simulink model "adaptive_t1"  (R2017a)
settings: Solver=FixedStepAuto  StartTime=0.0  StopTime=8  FixedStep=0.001  RelTol=1e-3
libraries: fuzblock x2
settings Model: Creator=Chaohua Zhao  LastModifiedBy=Chaohua Zhao

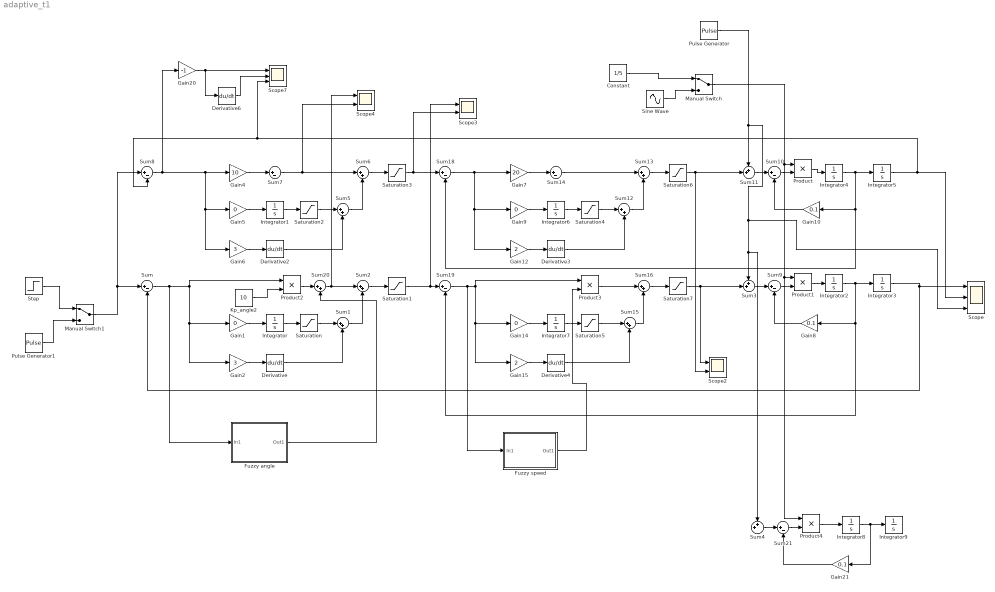
== system adaptive_t1 ==
  Constant : Constant  Value=1/5
  Derivative{,2..4,6} (5 alike) : Derivative
  "Fuzzy angle " : Subsystem
  Fuzzy speed : Subsystem
  Gain{1,5,9,14} (4 alike) : Gain  Gain=0
  Gain10 : Gain  Gain=0.1
  Gain12 : Gain  Gain=2
  Gain15 : Gain  Gain=2
  Gain2 : Gain  Gain=3
  Gain20 : Gain  Gain=-1
  Gain21 : Gain  Gain=0.1
  Gain4 : Gain  Gain=10
  Gain6 : Gain  Gain=3
  Gain7 : Gain  Gain=20
  Gain8 : Gain  Gain=0.1
  Integrator{,1..9} (10 alike) : Integrator
  Kp_angle2 : Constant  Value=10
  Manual Switch : ManualSwitch
  Manual Switch1 : ManualSwitch
  Product{,1..4} (5 alike) : Product
  Pulse Generator : DiscretePulseGenerator  PulseType=Time based  Amplitude=0.1  Period=3  PulseWidth=4  PhaseDelay=5
  Pulse Generator1 : DiscretePulseGenerator  PulseType=Time based  Period=15  PulseWidth=50
  Saturation{,2,4..5} (4 alike) : Saturate
  Saturation1 : Saturate  UpperLimit=100  LowerLimit=-100
  Saturation3 : Saturate  UpperLimit=100  LowerLimit=-100
  Saturation6 : Saturate  UpperLimit=10  LowerLimit=-10
  Saturation7 : Saturate  UpperLimit=10  LowerLimit=-10
  Scope : Scope  NumInputPorts=3
  Scope2 : Scope  NumInputPorts=2
  Scope3 : Scope  NumInputPorts=2
  Scope4 : Scope  NumInputPorts=2
  Scope7 : Scope  NumInputPorts=3
  Sine Wave : Sin  Amplitude=0.4  Bias=0.5  SampleTime=0
  Step : Step  Time=0  After=3  SampleTime=0
  Sum{,7..10,14,18..19,21} (9 alike) : Sum  Inputs=|+-
  Sum{1..2,5..6,12..13,15..16,20} (9 alike) : Sum  Inputs=|++
  Sum11 : Sum  Inputs=++|
  Sum3 : Sum  Inputs=++|
  Sum4 : Sum  Inputs=++|
  wires:
  Integrator3/1 -> Scope/1, Sum/2
  Sum/1 -> "Fuzzy angle "/1(In1), Product2/1, Gain1/1, Gain2/1
  Saturation/1 -> Sum1/1
  Integrator/1 -> Saturation/1
  Gain1/1 -> Integrator/1
  Gain2/1 -> Derivative/1
  Derivative/1 -> Sum1/2
  Sum1/1 -> Sum2/2
  Sum2/1 -> Saturation1/1
  Sum7/1 -> Scope4/2, Sum6/1
  Gain4/1 -> Sum7/1
  Sum6/1 -> Saturation3/1
  Sum5/1 -> Sum6/2
  Derivative2/1 -> Sum5/2
  Gain6/1 -> Derivative2/1
  Gain5/1 -> Integrator1/1
  Integrator1/1 -> Saturation2/1
  Saturation2/1 -> Sum5/1
  Sum8/1 -> Gain20/1, Gain4/1, Gain5/1, Gain6/1
  Integrator5/1 -> Scope7/3, Sum8/2, Scope/2
  Integrator2/1 -> Sum19/2, Gain8/1, Integrator3/1
  Sum3/1 -> Sum9/1
  Integrator4/1 -> Integrator5/1, Sum18/2, Gain10/1
  Sum11/1 -> Sum10/1
  Pulse Generator/1 -> Scope/3, Sum4/1, Sum3/1, Sum11/1
  Sum10/1 -> Product/2
  Product/1 -> Integrator4/1
  Sum9/1 -> Product1/2
  Product1/1 -> Integrator2/1
  Sine Wave/1 -> Manual Switch/2
  Constant/1 -> Manual Switch/1
  Manual Switch/1 -> Product1/1, Product4/1, Product/1
  Pulse Generator1/1 -> Manual Switch1/2
  Manual Switch1/1 -> Sum8/1, Sum/1
  Saturation4/1 -> Sum12/1
  Integrator6/1 -> Saturation4/1
  Gain9/1 -> Integrator6/1
  Gain12/1 -> Derivative3/1
  Derivative3/1 -> Sum12/2
  Sum12/1 -> Sum13/2
  Sum13/1 -> Saturation6/1
  Gain7/1 -> Sum14/1
  Sum14/1 -> Sum13/1
  Product3/1 -> Sum16/1
  Sum15/1 -> Sum16/2
  Derivative4/1 -> Sum15/2
  Gain15/1 -> Derivative4/1
  Gain14/1 -> Integrator7/1
  Integrator7/1 -> Saturation5/1
  Saturation5/1 -> Sum15/1
  Sum16/1 -> Saturation7/1
  Saturation6/1 -> Sum11/2, Scope2/2
  Saturation7/1 -> Sum3/2, Scope2/1
  Sum18/1 -> Gain12/1, Gain9/1, Gain7/1
  Saturation1/1 -> Scope3/1, Sum19/1
  Saturation3/1 -> Scope3/2, Sum18/1
  Step/1 -> Manual Switch1/1
  Sum19/1 -> Fuzzy speed/1(In1), Product3/1, Gain15/1, Gain14/1
  Product2/1 -> Sum20/1
  Sum20/1 -> Sum2/1, Scope4/1
  Kp_angle2/1 -> Product2/2
  Gain20/1 -> Derivative6/1, Scope7/1
  Derivative6/1 -> Scope7/2
  Product4/1 -> Integrator8/1
  Sum21/1 -> Product4/2
  Sum4/1 -> Sum21/1
  Integrator8/1 -> Gain21/1, Integrator9/1
  Gain8/1 -> Sum9/2
  Gain10/1 -> Sum10/2
  Gain21/1 -> Sum21/2
  "Fuzzy angle "/1(Out1) -> Sum20/2
  Fuzzy speed/1(Out1) -> Product3/2

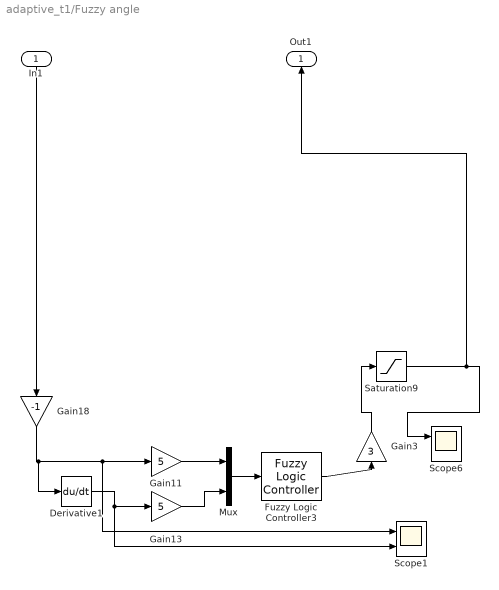
== system adaptive_t1/Fuzzy angle  ==
  In1 : Inport
  Derivative1 : Derivative
  Fuzzy Logic Controller3 : fuzblock/Fuzzy Logic  Controller  fis='Fuzzy_sug_t1.fis'
  Gain11 : Gain  Gain=5
  Gain13 : Gain  Gain=5
  Gain18 : Gain  Gain=-1
  Gain3 : Gain  Gain=3
  Mux : Mux  Inputs=2
  Saturation9 : Saturate  UpperLimit=100  LowerLimit=0
  Scope1 : Scope  NumInputPorts=2
  Scope6 : Scope  NumInputPorts=2
  Out1 : Outport
  wires:
  Derivative1/1 -> Gain13/1, Scope1/2
  Fuzzy Logic Controller3/1 -> Gain3/1
  Mux/1 -> Fuzzy Logic Controller3/1
  Gain18/1 -> Derivative1/1, Gain11/1, Scope1/1
  Gain11/1 -> Mux/1
  Gain3/1 -> Saturation9/1
  Saturation9/1 -> Out1/1, Scope6/1
  Gain13/1 -> Mux/2
  In1/1 -> Gain18/1

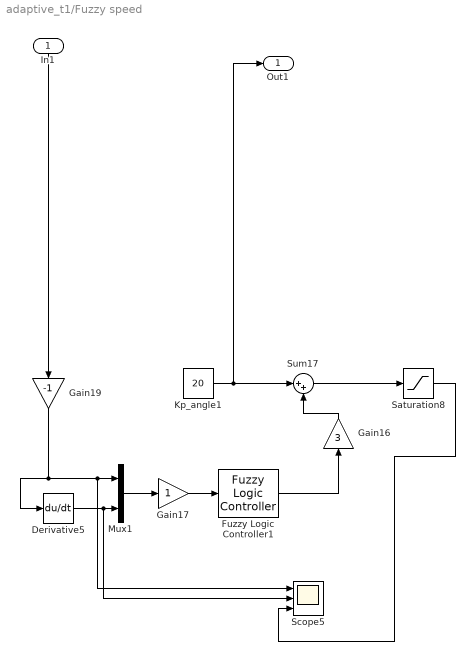
== system adaptive_t1/Fuzzy speed ==
  In1 : Inport
  Derivative5 : Derivative
  Fuzzy Logic Controller1 : fuzblock/Fuzzy Logic  Controller  fis='Fuzzy_t1.fis'
  Gain16 : Gain  Gain=3
  Gain17 : Gain
  Gain19 : Gain  Gain=-1
  Kp_angle1 : Constant  Value=20
  Mux1 : Mux  Inputs=2
  Saturation8 : Saturate  UpperLimit=100  LowerLimit=0
  Scope5 : Scope  NumInputPorts=3
  Sum17 : Sum  Inputs=|++
  Out1 : Outport
  wires:
  Derivative5/1 -> Scope5/2, Mux1/2
  Mux1/1 -> Gain17/1
  Fuzzy Logic Controller1/1 -> Gain16/1
  Gain16/1 -> Sum17/2
  Gain17/1 -> Fuzzy Logic Controller1/1
  Kp_angle1/1 -> Out1/1, Sum17/1
  Sum17/1 -> Saturation8/1
  Gain19/1 -> Derivative5/1, Scope5/1, Mux1/1
  Saturation8/1 -> Scope5/3
  In1/1 -> Gain19/1
